simulink model "rsa_mwr2mm_core"  (R2021b)
settings: Solver=VariableStepAuto  StartTime=0.0  StopTime=simulation_time  RelTol=1e-3
values from neighbouring files (symbols this model uses):
  E = fi(hex2dec("4741"),0,max_n_bit,0)    [mwr2mm_init.m]    (also in rsa_mwr2mm_init.m)
  K = fi(mod((4)^max_n_bit,double(N)),0,max_n_bit,0)    [mwr2mm_init.m]    (also in rsa_mwr2mm_init.m)
  M = fi(hex2dec("2f76"),0,max_n_bit,0)    [mwr2mm_init.m]    (also in rsa_mwr2mm_init.m)
  max_n_bit = 16    [mwr2mm_init.m]    (also in rsa_mwr2mm_init.m)
  N = fi(hex2dec("8167"),0,max_n_bit,0)    [mwr2mm_init.m]    (also in rsa_mwr2mm_init.m)
  number_of_pe = ceil((max_n_bit+1)/word_length)    [mwr2mm_init.m]    (also in rsa_mwr2mm_init.m)
  ts = 1/fs    (= 4e-09)    [mwr2mm_init.m]    (also in rsa_mwr2mm_init.m)
  word_length = 4    [mwr2mm_init.m]    (also in rsa_mwr2mm_init.m)
libraries: xbsIndex_r4 x206
(part 2 of 2)

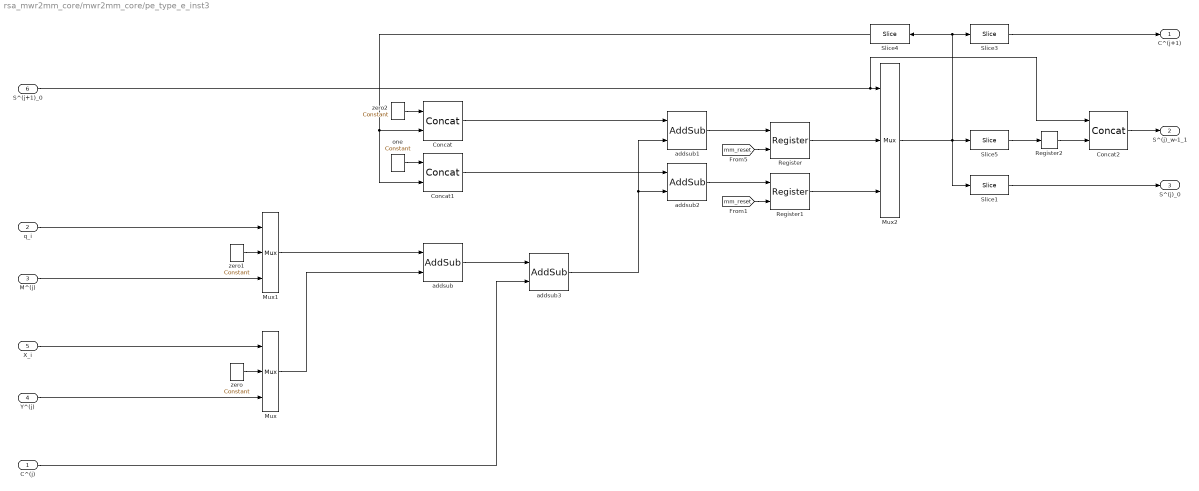
== system rsa_mwr2mm_core/mwr2mm_core/pe_type_e_inst3 ==
  C^(j) : Inport
  q_i : Inport  Port=2
  M^(j) : Inport  Port=3
  Y^(j) : Inport  Port=4
  X_i : Inport  Port=5
  S^(j+1)_0 : Inport  Port=6
  Concat : xbsIndex_r4/Concat  num_inputs=2  dbl_ovrd=off  block_type=concat
  Concat1 : xbsIndex_r4/Concat  num_inputs=2  dbl_ovrd=off  block_type=concat
  Concat2 : xbsIndex_r4/Concat  num_inputs=2  dbl_ovrd=off  block_type=concat
  Mux : xbsIndex_r4/Mux  inputs=2  en=off  latency=0  precision=Full  arith_type=Unsigned  n_bits=16  bin_pt=14  quantization=Truncate  overflow=Wrap  dbl_ovrd=off  block_type=mux
  Mux1 : xbsIndex_r4/Mux  inputs=2  en=off  latency=0  precision=Full  arith_type=Unsigned  n_bits=16  bin_pt=14  quantization=Truncate  overflow=Wrap  dbl_ovrd=off  block_type=mux
  Mux2 : xbsIndex_r4/Mux  inputs=2  en=off  latency=0  precision=Full  arith_type=Unsigned  n_bits=16  bin_pt=14  quantization=Truncate  overflow=Wrap  dbl_ovrd=off  block_type=mux
  Register : xbsIndex_r4/Register  init=0  rst=on  en=off  dbl_ovrd=off  block_type=register
  Register1 : xbsIndex_r4/Register  init=0  rst=on  en=off  dbl_ovrd=off  block_type=register
  Register2 : xbsIndex_r4/Register  init=0  rst=off  en=off  dbl_ovrd=off  block_type=register
  Slice1 : xbsIndex_r4/Slice  nbits=word_length-1  boolean_output=on  mode=Lower Bit Location + Width  bit1=0  base1=MSB of Input  bit0=0  base0=LSB of Input  dbl_ovrd=off  block_type=slice
  Slice3 : xbsIndex_r4/Slice  nbits=2  boolean_output=off  mode=Lower Bit Location + Width  bit1=0  base1=MSB of Input  bit0=word_length  base0=LSB of Input  dbl_ovrd=off  block_type=slice
  Slice4 : xbsIndex_r4/Slice  nbits=word_length-1  boolean_output=off  mode=Lower Bit Location + Width  bit1=0  base1=MSB of Input  bit0=1  base0=LSB of Input  dbl_ovrd=off  block_type=slice
  Slice5 : xbsIndex_r4/Slice  nbits=word_length-1  boolean_output=off  mode=Lower Bit Location + Width  bit1=0  base1=MSB of Input  bit0=1  base0=LSB of Input  dbl_ovrd=off  block_type=slice
  addsub : xbsIndex_r4/AddSub  mode=Addition  use_carryin=off  use_carryout=off  en=off  latency=0  precision=User Defined  arith_type=Unsigned  n_bits=word_length+1  bin_pt=0  quantization="Round  (unbiased: +/- Inf)"  overflow=Saturate  use_behavioral_HDL=off  hw_selection=Fabric  pipelined=on  dbl_ovrd=off  block_type=addsub
  addsub1 : xbsIndex_r4/AddSub  mode=Addition  use_carryin=off  use_carryout=off  en=off  latency=0  precision=User Defined  arith_type=Unsigned  n_bits=word_length+2  bin_pt=0  quantization="Round  (unbiased: +/- Inf)"  overflow=Saturate  use_behavioral_HDL=off  hw_selection=Fabric  pipelined=on  dbl_ovrd=off  block_type=addsub
  addsub2 : xbsIndex_r4/AddSub  mode=Addition  use_carryin=off  use_carryout=off  en=off  latency=0  precision=User Defined  arith_type=Unsigned  n_bits=word_length+2  bin_pt=0  quantization="Round  (unbiased: +/- Inf)"  overflow=Saturate  use_behavioral_HDL=off  hw_selection=Fabric  pipelined=on  dbl_ovrd=off  block_type=addsub
  addsub3 : xbsIndex_r4/AddSub  mode=Addition  use_carryin=off  use_carryout=off  en=off  latency=0  precision=User Defined  arith_type=Unsigned  n_bits=word_length+2  bin_pt=0  quantization="Round  (unbiased: +/- Inf)"  overflow=Saturate  use_behavioral_HDL=off  hw_selection=Fabric  pipelined=on  dbl_ovrd=off  block_type=addsub
  one : xbsIndex_r4/Constant  const=1  gui_display_data_type=Fixed-point  arith_type=Unsigned  n_bits=1  bin_pt=0  preci_type=Single  exp_width=8  frac_width=24  explicit_period=off  period=1  equ=P=C  opselect=C  inp2=PCIN>>17  opr=+  inp1=P  carry=CIN  dbl_ovrd=off  block_type=constant
  zero : xbsIndex_r4/Constant  const=0  gui_display_data_type=Fixed-point  arith_type=Unsigned  n_bits=1  bin_pt=0  preci_type=Single  exp_width=8  frac_width=24  explicit_period=off  period=1  equ=P=C  opselect=C  inp2=PCIN>>17  opr=+  inp1=P  carry=CIN  dbl_ovrd=off  block_type=constant
  zero1 : xbsIndex_r4/Constant  const=0  gui_display_data_type=Fixed-point  arith_type=Unsigned  n_bits=1  bin_pt=0  preci_type=Single  exp_width=8  frac_width=24  explicit_period=off  period=1  equ=P=C  opselect=C  inp2=PCIN>>17  opr=+  inp1=P  carry=CIN  dbl_ovrd=off  block_type=constant
  zero2 : xbsIndex_r4/Constant  const=0  gui_display_data_type=Fixed-point  arith_type=Unsigned  n_bits=1  bin_pt=0  preci_type=Single  exp_width=8  frac_width=24  explicit_period=off  period=1  equ=P=C  opselect=C  inp2=PCIN>>17  opr=+  inp1=P  carry=CIN  dbl_ovrd=off  block_type=constant
  C^(j+1) : Outport
  S^(j)_w-1_1 : Outport  Port=2
  S^(j)_0 : Outport  Port=3
  wires:
  Slice5/1 -> Register2/1
  Register2/1 -> Concat2/2
  S^(j+1)_0/1 -> Mux2/1, Concat2/1
  Slice4/1 -> Concat1/2, Concat/2
  [mm_reset] -> Register1/2
  [mm_reset] -> Register/2
  Slice1/1 -> S^(j)_0/1
  C^(j)/1 -> addsub3/2
  addsub/1 -> addsub3/1
  Concat2/1 -> S^(j)_w-1_1/1
  q_i/1 -> Mux1/1
  Mux2/1 -> Slice3/1, Slice4/1, Slice1/1, Slice5/1
  addsub2/1 -> Register1/1
  addsub1/1 -> Register/1
  addsub3/1 -> addsub2/2, addsub1/2
  Concat1/1 -> addsub2/1
  Concat/1 -> addsub1/1
  one/1 -> Concat1/1
  zero2/1 -> Concat/1
  Mux1/1 -> addsub/1
  Mux/1 -> addsub/2
  zero1/1 -> Mux1/2
  Y^(j)/1 -> Mux/3
  zero/1 -> Mux/2
  M^(j)/1 -> Mux1/3
  X_i/1 -> Mux/1
  Register/1 -> Mux2/2
  Register1/1 -> Mux2/3
  Slice3/1 -> C^(j+1)/1

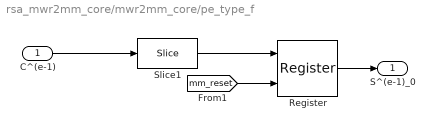
== system rsa_mwr2mm_core/mwr2mm_core/pe_type_f ==
  C^(e-1) : Inport
  Register : xbsIndex_r4/Register  init=0  rst=on  en=off  dbl_ovrd=off  block_type=register
  Slice1 : xbsIndex_r4/Slice  nbits=word_length-1  boolean_output=on  mode=Lower Bit Location + Width  bit1=0  base1=MSB of Input  bit0=0  base0=LSB of Input  dbl_ovrd=off  block_type=slice
  S^(e-1)_0 : Outport
  wires:
  [mm_reset] -> Register/2
  C^(e-1)/1 -> Slice1/1
  Slice1/1 -> Register/1
  Register/1 -> S^(e-1)_0/1

== system rsa_mwr2mm_core/mwr2mm_core/rising_edge ==
  input : Inport
  Inverter1 : xbsIndex_r4/Inverter  en=off  latency=1  dbl_ovrd=off  block_type=inv
  Logical1 : xbsIndex_r4/Logical  logical_function=AND  inputs=2  en=off  latency=0  precision=Full  arith_type=Unsigned  n_bits=16  bin_pt=0  align_bp=on  dbl_ovrd=off  block_type=logical
  redge : Outport
  wires:
  Inverter1/1 -> Logical1/2
  input/1 -> Inverter1/1, Logical1/1
  Logical1/1 -> redge/1

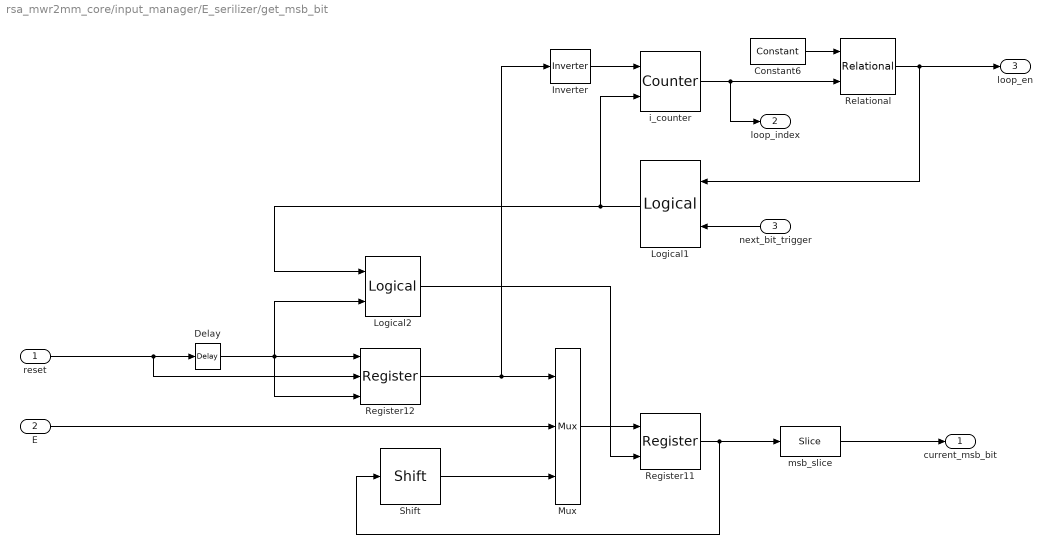
== system rsa_mwr2mm_core/input_manager/E_serilizer/get_msb_bit ==
  reset : Inport
  E : Inport  Port=2
  next_bit_trigger : Inport  Port=3
  Constant6 : xbsIndex_r4/Constant  const=max_n_bit-1  gui_display_data_type=Fixed-point  arith_type=Unsigned  n_bits=ceil(log2(max_n_bit))  bin_pt=0  preci_type=Single  exp_width=8  frac_width=24  explicit_period=on  period=ts  equ=P=C  opselect=C  inp2=PCIN>>17  opr=+  inp1=P  carry=CIN  dbl_ovrd=off  block_type=constant
  Delay : xbsIndex_r4/Delay  rst=off  infoeditControl=Selection of Reset will increase slice count due to use of real FFs and instead of SRLs  en=off  latency=5  reg_retiming=off  dbl_ovrd=off  block_type=delay
  Inverter : xbsIndex_r4/Inverter  en=off  latency=0  dbl_ovrd=off  block_type=inv
  Logical1 : xbsIndex_r4/Logical  logical_function=AND  inputs=2  en=off  latency=1  precision=Full  arith_type=Unsigned  n_bits=16  bin_pt=0  align_bp=on  dbl_ovrd=off  block_type=logical
  Logical2 : xbsIndex_r4/Logical  logical_function=OR  inputs=2  en=off  latency=0  precision=Full  arith_type=Unsigned  n_bits=16  bin_pt=0  align_bp=on  dbl_ovrd=off  block_type=logical
  Mux : xbsIndex_r4/Mux  inputs=2  en=off  latency=0  precision=Full  arith_type=Unsigned  n_bits=16  bin_pt=14  quantization=Truncate  overflow=Wrap  dbl_ovrd=off  block_type=mux
  Register11 : xbsIndex_r4/Register  init=0  rst=off  en=on  dbl_ovrd=off  block_type=register
  Register12 : xbsIndex_r4/Register  init=0  rst=on  en=on  dbl_ovrd=off  block_type=register
  Relational : xbsIndex_r4/Relational  mode=a>=b  op_type=Bool  en=off  latency=0  dbl_ovrd=off  block_type=relational
  Shift : xbsIndex_r4/Shift  shift_dir=Left  shift_bits=1  en=off  latency=0  precision=Full  arith_type="Signed  (2's comp)"  n_bits=16  bin_pt=14  quantization=Truncate  overflow=Wrap  dbl_ovrd=off  block_type=shift
  i_counter : xbsIndex_r4/Counter  cnt_type=Free Running  cnt_to=Inf  operation=Up  start_count=0  cnt_by_val=1  arith_type=Unsigned  n_bits=ceil(log2(max_n_bit))+1  bin_pt=0  load_pin=off  rst=on  en=on  explicit_period=off  period=1  use_behavioral_HDL=off  implementation=Fabric  dbl_ovrd=off  block_type=counter
  msb_slice : xbsIndex_r4/Slice  nbits=1  boolean_output=on  mode=Upper Bit Location + Width  bit1=0  base1=MSB of Input  bit0=0  base0=LSB of Input  dbl_ovrd=off  block_type=slice
  current_msb_bit : Outport
  loop_index : Outport  Port=2
  loop_en : Outport  Port=3
  wires:
  Register11/1 -> Shift/1, msb_slice/1
  i_counter/1 -> loop_index/1, Relational/2
  Register12/1 -> Inverter/1, Mux/1
  Logical1/1 -> Logical2/1, i_counter/2
  Shift/1 -> Mux/3
  Mux/1 -> Register11/1
  E/1 -> Mux/2
  next_bit_trigger/1 -> Logical1/2
  Inverter/1 -> i_counter/1
  reset/1 -> Register12/2, Delay/1
  Delay/1 -> Register12/3, Logical2/2, Register12/1
  Relational/1 -> loop_en/1, Logical1/1
  Logical2/1 -> Register11/2
  msb_slice/1 -> current_msb_bit/1
  Constant6/1 -> Relational/1

== system rsa_mwr2mm_core/input_manager/E_serilizer/rising_edge ==
  input : Inport
  Inverter1 : xbsIndex_r4/Inverter  en=off  latency=1  dbl_ovrd=off  block_type=inv
  Logical1 : xbsIndex_r4/Logical  logical_function=AND  inputs=2  en=off  latency=0  precision=Full  arith_type=Unsigned  n_bits=16  bin_pt=0  align_bp=on  dbl_ovrd=off  block_type=logical
  redge : Outport
  wires:
  Inverter1/1 -> Logical1/2
  input/1 -> Inverter1/1, Logical1/1
  Logical1/1 -> redge/1

== system rsa_mwr2mm_core/input_manager/E_serilizer/rising_edge1 ==
  input : Inport
  Inverter1 : xbsIndex_r4/Inverter  en=off  latency=1  dbl_ovrd=off  block_type=inv
  Logical1 : xbsIndex_r4/Logical  logical_function=AND  inputs=2  en=off  latency=0  precision=Full  arith_type=Unsigned  n_bits=16  bin_pt=0  align_bp=on  dbl_ovrd=off  block_type=logical
  redge : Outport
  wires:
  Logical1/1 -> redge/1
  input/1 -> Logical1/1, Inverter1/1
  Inverter1/1 -> Logical1/2

== system rsa_mwr2mm_core/input_manager/E_serilizer/rising_edge2 ==
  input : Inport
  Inverter1 : xbsIndex_r4/Inverter  en=off  latency=1  dbl_ovrd=off  block_type=inv
  Logical1 : xbsIndex_r4/Logical  logical_function=AND  inputs=2  en=off  latency=0  precision=Full  arith_type=Unsigned  n_bits=16  bin_pt=0  align_bp=on  dbl_ovrd=off  block_type=logical
  redge : Outport
  wires:
  Inverter1/1 -> Logical1/2
  input/1 -> Inverter1/1, Logical1/1
  Logical1/1 -> redge/1
